simulink model "sToPosition2_th"  (R2018b)
settings: Solver=VariableStepAuto  StartTime=0.0  StopTime=10.0  RelTol=1e-3
libraries: courseFollow_cl x1
settings Model: Creator=James Reed  LastModifiedBy=James Reed

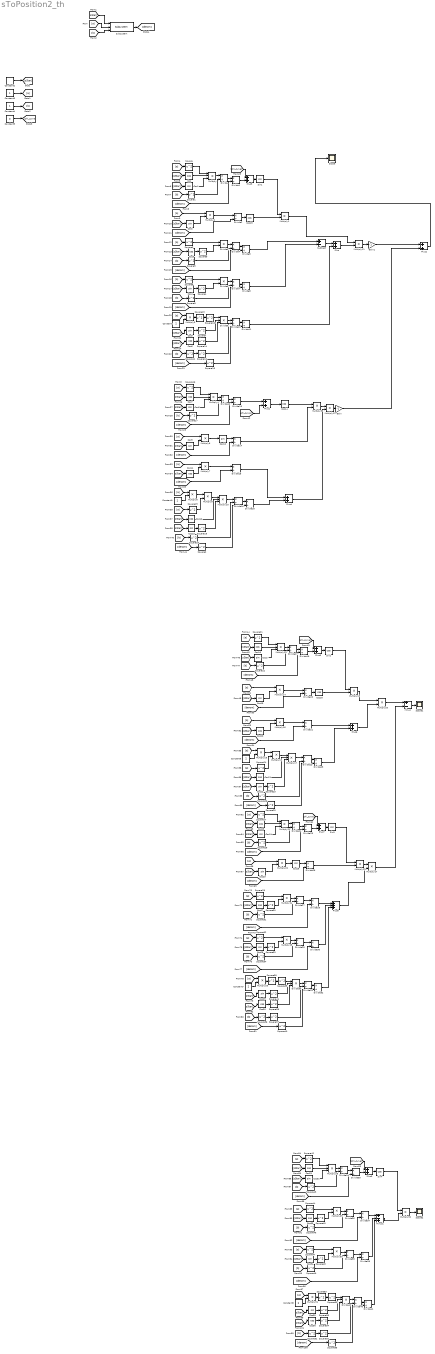
== system sToPosition2_th ==
  Constant{,1,6..8} (5 alike) : Constant  Value=2
  Constant2 : Constant  Value=3.1205
  Constant3 : Constant
  Constant4 : Constant
  Constant5 : Constant  Value=0
  Cos{,3,6..7,11..12,14..16,18,20..21,23,27,30..31,33,36} (18 alike) : Trigonometry  Operator=cos
  Cos{1..2,4..5,8..10,13,17,19,22,24..26,28..29,32,34..35} (19 alike) : Trigonometry
  Divide{,1..2,4..5,7..8,10..32,34..41} (38 alike) : Product  Inputs=*/
  Divide3 : Product  Inputs=**
  Divide33 : Product  Inputs=***
  Divide42 : Product  Inputs=***
  Divide6 : Product  Inputs=**
  Divide9 : Product  Inputs=***
  Gain : Gain  Gain=-1
  Gain1 : Gain  Gain=-1
  Minus : Sum  Inputs=+-
  Minus1 : Sum  Inputs=+-+
  Multiply{,4,10,13,17,21,28} (7 alike) : Product  Inputs=3
  Multiply{1..3,5..9,11..12,14..16,18..20,22..27,29..32} (26 alike) : Product
  Plus{,1..3,5..7,9} (8 alike) : Sum
  Plus4 : Sum  Inputs=2
  Plus8 : Sum  Inputs=+-+
  Scope : Scope
  Scope1 : Scope
  Scope2 : Scope
  Sin1 : Trigonometry
  Sin2 : Trigonometry  Operator=cos
  Sin3 : Trigonometry
  Sin4 : Trigonometry  Operator=cos
  Square{,1..56} (57 alike) : Math  Operator=square  SaturateOnIntegerOverflow=on
  Subsystem : courseFollow_cl/courseFollow/s_to_position (TODO)/Subsystem  SystemSampleTime=-1
  Subtract : Sum  Inputs=+-
  wires:
  Constant4/1 -> [b]
  Constant5/1 -> [phi_curve]
  Constant3/1 -> [a]
  Constant2/1 -> [sStar]
  [sStar] -> Subsystem/1
  [a] -> Subsystem/2
  Subsystem/1 -> [denom]
  [b] -> Subsystem/3
  Divide8/1 -> Subtract/2
  Divide7/1 -> Divide8/1
  [b] -> Square8/1
  [denom] -> Divide8/2
  Square8/1 -> Divide7/2
  Divide6/1 -> Divide7/1
  [a] -> Square6/1
  Constant1/1 -> Multiply8/2
  [a] -> Multiply8/1
  [sStar] -> Cos4/1
  Divide1/1 -> Plus3/2
  Gain1/1 -> Plus2/1
  Multiply1/1 -> Multiply11/1
  Multiply2/1 -> Divide2/1
  [phi_curve] -> Plus1/2
  Divide2/1 -> Cos15/1
  [a] -> Square19/1
  Multiply9/1 -> Multiply10/1
  Square19/1 -> Multiply9/2
  Multiply8/1 -> Multiply9/1
  [sStar] -> Cos13/1
  [sStar] -> Cos12/1
  Cos12/1 -> Multiply10/2
  Square18/1 -> Multiply10/3
  [denom] -> Square2/1
  Multiply11/1 -> Gain1/1
  Sin1/1 -> Multiply1/1
  Plus/1 -> Multiply11/2
  [b] -> Square1/1
  Square1/1 -> Divide/2
  [sStar] -> Cos1/1
  [sStar] -> Cos/1
  Cos1/1 -> Multiply/3
  Cos/1 -> Multiply/2
  Cos11/1 -> Multiply7/2
  [sStar] -> Cos11/1
  Cos3/1 -> Square9/1
  Square20/1 -> Divide16/2
  Multiply10/1 -> Divide16/1
  [b] -> Square20/1
  Square5/1 -> Divide4/2
  Subtract/1 -> Plus/1
  Multiply/1 -> Divide/1
  [a] -> Square3/1
  Cos6/1 -> Square14/1
  Square11/1 -> Square12/1
  [a] -> Multiply3/1
  Divide/1 -> Divide1/1
  [b] -> Square5/1
  [denom] -> Divide15/2
  Plus1/1 -> Cos14/1
  Square9/1 -> Divide3/2
  Square3/1 -> Divide3/1
  [sStar] -> Cos3/1
  [a] -> Multiply6/1
  Cos4/1 -> Square4/1
  [denom] -> Square15/1
  [denom] -> Divide1/2
  Divide14/1 -> Multiply5/2
  Square10/1 -> Divide9/1
  Divide16/1 -> Divide18/1
  Cos9/1 -> Multiply6/2
  Divide9/1 -> Divide10/1
  Cos15/1 -> Multiply1/2
  [sStar] -> Cos5/1
  Divide3/1 -> Divide4/1
  [a] -> Multiply2/1
  Divide15/1 -> Plus4/1
  Divide13/1 -> Plus1/1
  [denom] -> Divide2/2
  Square14/1 -> Divide9/3
  Divide5/1 -> Subtract/1
  [sStar] -> Cos2/1
  Plus4/1 -> Multiply12/2
  [a] -> Multiply7/1
  Divide18/1 -> Plus4/2
  Plus3/1 -> Sin1/1
  [phi_curve] -> Plus3/1
  Square/1 -> Multiply/1
  Square12/1 -> Divide10/2
  Divide11/1 -> Plus/2
  Multiply3/1 -> Square13/1
  Divide4/1 -> Divide5/1
  Cos2/1 -> Multiply2/2
  Square15/1 -> Divide11/2
  Cos5/1 -> Square7/1
  [sStar] -> Cos9/1
  Square13/1 -> Square10/1
  [denom] -> Divide14/2
  Square4/1 -> Divide6/2
  [denom] -> Divide5/2
  Cos13/1 -> Square18/1
  Cos10/1 -> Divide14/1
  Square2/1 -> Divide18/2
  [b] -> Square11/1
  Square7/1 -> Divide9/2
  [sStar] -> Cos7/1
  [sStar] -> Cos6/1
  Cos7/1 -> Multiply4/2
  Multiply7/1 -> Divide15/1
  Square6/1 -> Divide6/1
  Multiply5/1 -> Multiply12/1
  Square17/1 -> Divide12/2
  Multiply12/1 -> Gain/1
  [sStar] -> Cos8/1
  [denom] -> Divide13/2
  Cos14/1 -> Multiply5/1
  [b] -> Square17/1
  Cos8/1 -> Multiply4/3
  Divide10/1 -> Divide11/1
  Constant/1 -> Multiply3/2
  [a] -> Square/1
  [a] -> Square16/1
  Multiply6/1 -> Cos10/1
  Divide12/1 -> Divide13/1
  Gain/1 -> Plus2/2
  Square16/1 -> Multiply4/1
  Multiply4/1 -> Divide12/1
  Plus2/1 -> Scope/1
  Multiply14/1 -> Divide20/1
  Cos19/1 -> Multiply14/2
  [a] -> Multiply14/1
  [sStar] -> Cos19/1
  [denom] -> Divide20/2
  Sin3/1 -> Multiply23/1
  Plus5/1 -> Sin2/1
  [a] -> Square21/1
  Square21/1 -> Multiply13/1
  [denom] -> Divide19/2
  Multiply13/1 -> Divide17/1
  Divide19/1 -> Plus5/2
  Cos17/1 -> Multiply13/3
  [sStar] -> Cos16/1
  [sStar] -> Cos17/1
  Square22/1 -> Divide17/2
  [sStar] -> Cos20/1
  [b] -> Square34/1
  Square33/1 -> Multiply25/2
  [denom] -> Divide30/2
  Cos28/1 -> Square33/1
  Square32/1 -> Multiply25/1
  Divide29/1 -> Divide30/1
  Square34/1 -> Divide29/2
  [sStar] -> Cos28/1
  Square29/1 -> Multiply24/1
  Divide32/1 -> Plus8/3
  Divide27/1 -> Divide28/1
  Cos27/1 -> Square30/1
  Multiply15/1 -> Multiply20/1
  [sStar] -> Cos27/1
  [a] -> Square29/1
  [phi_curve] -> Plus5/1
  Multiply23/1 -> Multiply27/1
  Multiply20/1 -> Minus/1
  Multiply27/1 -> Minus/2
  Multiply22/1 -> Cos26/1
  [denom] -> Divide21/2
  Constant6/1 -> Multiply18/2
  [a] -> Multiply18/1
  Cos22/1 -> Square23/1
  Multiply16/1 -> Divide21/1
  Multiply19/1 -> Multiply17/1
  Square25/1 -> Divide23/2
  Divide22/1 -> Divide23/1
  Square26/1 -> Divide22/2
  Cos21/1 -> Multiply17/2
  Divide20/1 -> Cos18/1
  [sStar] -> Cos22/1
  [a] -> Square24/1
  [sStar] -> Cos25/1
  Square31/1 -> Divide27/2
  [b] -> Square22/1
  Square23/1 -> Multiply17/3
  Square41/1 -> Divide33/2
  Multiply18/1 -> Multiply19/1
  Square24/1 -> Multiply19/2
  Cos29/1 -> Square41/1
  [a] -> Multiply26/1
  [denom] -> Divide26/2
  Square38/1 -> Square35/1
  [sStar] -> Cos29/1
  [b] -> Square36/1
  Square36/1 -> Square37/1
  [denom] -> Square40/1
  Constant7/1 -> Multiply26/2
  Square37/1 -> Divide31/2
  Multiply26/1 -> Square38/1
  Divide26/1 -> Multiply23/2
  Cos26/1 -> Divide26/1
  [a] -> Square32/1
  Square39/1 -> Divide33/3
  Square40/1 -> Divide32/2
  Cos20/1 -> Multiply16/2
  Divide21/1 -> Plus6/1
  Cos16/1 -> Multiply13/2
  Plus8/1 -> Multiply27/2
  Multiply24/1 -> Divide27/1
  Divide33/1 -> Divide31/1
  Divide28/1 -> Plus8/1
  [denom] -> Square25/1
  Cos18/1 -> Multiply15/2
  Sin2/1 -> Multiply15/1
  [a] -> Multiply16/1
  Divide24/1 -> Divide25/1
  [b] -> Square26/1
  [a] -> Multiply22/1
  [a] -> Square27/1
  Plus7/1 -> Sin3/1
  [sStar] -> Cos21/1
  Square30/1 -> Multiply24/2
  [sStar] -> Cos30/1
  [b] -> Square31/1
  Square35/1 -> Divide33/1
  [denom] -> Divide25/2
  Square28/1 -> Divide24/2
  Divide17/1 -> Divide19/1
  [sStar] -> Cos23/1
  Cos23/1 -> Multiply21/2
  Multiply17/1 -> Divide22/1
  [sStar] -> Cos24/1
  Square27/1 -> Multiply21/1
  Plus6/1 -> Multiply20/2
  Divide25/1 -> Plus7/2
  Cos30/1 -> Square39/1
  Divide31/1 -> Divide32/1
  [b] -> Square28/1
  Multiply21/1 -> Divide24/1
  Divide30/1 -> Plus8/2
  [phi_curve] -> Plus7/1
  Divide23/1 -> Plus6/2
  Cos25/1 -> Multiply22/2
  Multiply25/1 -> Divide29/1
  [denom] -> Divide28/2
  Cos24/1 -> Multiply21/3
  Minus/1 -> Scope1/1
  Divide37/1 -> Minus1/1
  [b] -> Square46/1
  [denom] -> Divide37/2
  Square45/1 -> Multiply29/2
  Square46/1 -> Divide36/2
  Square44/1 -> Multiply29/1
  [sStar] -> Cos31/1
  Square43/1 -> Divide34/2
  Cos33/1 -> Square45/1
  [sStar] -> Cos32/1
  Cos32/1 -> Multiply28/3
  Cos31/1 -> Multiply28/2
  Divide35/1 -> Plus9/2
  Square42/1 -> Multiply28/1
  Plus9/1 -> Sin4/1
  Cos36/1 -> Square54/1
  Square50/1 -> Divide42/1
  Square54/1 -> Divide42/3
  Divide42/1 -> Divide40/1
  Divide40/1 -> Divide41/1
  [b] -> Square43/1
  [sStar] -> Cos35/1
  Square53/1 -> Square50/1
  [a] -> Multiply31/1
  Cos35/1 -> Square56/1
  Square56/1 -> Divide42/2
  [denom] -> Square55/1
  [denom] -> Divide35/2
  [sStar] -> Cos33/1
  Square51/1 -> Square52/1
  Multiply28/1 -> Divide34/1
  [b] -> Square51/1
  [a] -> Square42/1
  Square52/1 -> Divide40/2
  Multiply31/1 -> Square53/1
  [sStar] -> Cos36/1
  Minus1/1 -> Multiply32/2
  Square48/1 -> Multiply30/2
  Constant8/1 -> Multiply31/2
  Square47/1 -> Multiply30/1
  [phi_curve] -> Plus9/1
  Square49/1 -> Divide38/2
  Divide38/1 -> Divide39/1
  [a] -> Square47/1
  Multiply29/1 -> Divide36/1
  [denom] -> Divide39/2
  Divide41/1 -> Minus1/3
  [b] -> Square49/1
  [sStar] -> Cos34/1
  Square55/1 -> Divide41/2
  Divide34/1 -> Divide35/1
  [a] -> Square44/1
  Sin4/1 -> Multiply32/1
  Divide36/1 -> Divide37/1
  Cos34/1 -> Square48/1
  Multiply30/1 -> Divide38/1
  Divide39/1 -> Minus1/2
  Multiply32/1 -> Scope2/1
